simulink model "HANcoder_E407_TTA_Controller_v3_2"  (R2018b)
settings: Solver=FixedStepDiscrete  StartTime=0.0  StopTime=1  FixedStep=0.01  RelTol=1e-3
PreLoadFcn:
  | librarySetup
  | eval([bdroot,'_startup']) %Calling [modelName]_startup.m
undefined symbols (not defined in the file): A0, A1, A2, A3, A4, Backup_Board, basic_cycle_duration_bc0, basic_cycle_duration_bc1, comm_delay_estimation1, comm_delay_estimation2, COMM_Period, COMM_Phase1, COMM_Phase2, COMM_Phase_init1, COMM_Phase_init2, COMP_duration, CON2, CON4, Controller1_Board, Controller2_Board, Controller3_Board, D10, D12, D13, D8, D9, delta_a_set, delta_f_set, delta_max, delta_min, delta_precision, e_width, frequency_IRQ, HANtuneOverride, hardware_granularity, I_a, I_f, idle_time_init, Input_Gen_Board, LA_Clock_Gr, LA_COMM_dly, LA_COMM_Err, LA_E_Desync, LA_MEX_Flag, LA_Task_Act, m_v, Master_Role, matrix_cycle_duration, matrix_rows, max_desync, max_num_msgs_CAN1, max_num_msgs_CAN2, min_desync, OutControl1_ID, OutControl2_ID, OutEmulator_ID, R_al, R_ar, R_fl, R_fr ... (+80)
libraries: hdlsllib x434, HANcoder_STM32_Target x28, simulink x3, simulink_extras x1
(part 13 of 31)

== system HANcoder_E407_TTA_Controller_v3_2/HANcoder STM32 Target - E407-STM32 algorithm/TTA CAN System/TTA System/Matrix Cycle Manager/Controller Matrix Cycle/controller basic cycle 1/COMP Task - Calculate Speed/Calculate speed ==
  note: Torque range: [tau_min, tau_max]
  note: Local variables
  note: Logic Analyzer - DEBUG
      | LT Update COMP task
      | activation
  note: Logic Analyzer - DEBUG
  Enable : EnablePort
  Constant1 : Constant  Priority=28  OutDataTypeStr=boolean
  Data Store Memory43 : DataStoreMemory  DataStoreName=v_ctreff  ReadBeforeWriteMsg=warning  WriteAfterWriteMsg=warning  WriteAfterReadMsg=warning  ShowAdditionalParam=off
  Data Store Memory44 : DataStoreMemory  DataStoreName=speed_error_prev  ReadBeforeWriteMsg=warning  WriteAfterWriteMsg=warning  WriteAfterReadMsg=warning  ShowAdditionalParam=off
  Data Store Memory46 : DataStoreMemory  DataStoreName=speed_derivative  ReadBeforeWriteMsg=warning  WriteAfterWriteMsg=warning  WriteAfterReadMsg=warning  ShowAdditionalParam=off
  Data Store Read : DataStoreRead  DataStoreName=theta_dot_fr
  Data Store Read1 : DataStoreRead  DataStoreName=theta_dot_fl
  Data Store Read10 : DataStoreRead  DataStoreName=speed_integral
  Data Store Read11 : DataStoreRead  DataStoreName=speed_derivative
  Data Store Read12 : DataStoreRead  DataStoreName=torque_fr_out
  Data Store Read13 : DataStoreRead  DataStoreName=v_ctreff
  Data Store Read14 : DataStoreRead  DataStoreName=torque_fl_out
  Data Store Read15 : DataStoreRead  DataStoreName=torque_ar_out
  Data Store Read16 : DataStoreRead  DataStoreName=torque_al_out
  Data Store Read2 : DataStoreRead  DataStoreName=theta_dot_ar
  Data Store Read3 : DataStoreRead  DataStoreName=theta_dot_al
  Data Store Read4 : DataStoreRead  DataStoreName=v_est
  Data Store Read5 : DataStoreRead  DataStoreName=v_set_stored
  Data Store Read6 : DataStoreRead  DataStoreName=speed_error_prev
  Data Store Read7 : DataStoreRead  DataStoreName=rx_data_incr_time
  Data Store Read9 : DataStoreRead  DataStoreName=speed_integral
  Data Store Write : DataStoreWrite  Priority=1  DataStoreName=v_est
  Data Store Write1 : DataStoreWrite  Priority=30  DataStoreName=speed_error_prev
  Data Store Write2 : DataStoreWrite  Priority=20  DataStoreName=speed_integral
  Data Store Write3 : DataStoreWrite  Priority=21  DataStoreName=speed_derivative
  Data Store Write4 : DataStoreWrite  Priority=40  DataStoreName=v_ctreff
  Data Store Write5 : DataStoreWrite  Priority=51  DataStoreName=torque_fl_set
  Data Store Write6 : DataStoreWrite  Priority=50  DataStoreName=torque_fr_set
  Data Store Write7 : DataStoreWrite  Priority=52  DataStoreName=torque_ar_set
  Data Store Write8 : DataStoreWrite  Priority=53  DataStoreName=torque_al_set
  Data Store Write9 : DataStoreWrite  Priority=29  DataStoreName=Toggle_Pin_A0
  Derivative speed : Subsystem
  Gain : Gain  Gain=R_fr
  Gain1 : Gain  Gain=R_fl
  Gain2 : Gain  Gain=R_ar
  Gain3 : Gain  Gain=R_al
  Gain4 : Gain  Gain=1/4
  Gain5 : Gain  Gain=speed_k_p
  Gain6 : Gain  Gain=speed_k_i
  Gain7 : Gain  Gain=speed_k_d
  Integral speed : Subsystem
  Saturation{,1..3} (4 alike) : Saturate  UpperLimit=tau_max  LowerLimit=tau_min
  Saturation4 : Saturate  UpperLimit=speed_max  LowerLimit=speed_min
  Sum : Sum  Inputs=++++
  Sum1 : Sum  Priority=10  Inputs=+-
  Sum2 : Sum  Inputs=+++
  Sum{3..6} (4 alike) : Sum
  wires:
  Data Store Read/1 -> Gain/1
  Data Store Read1/1 -> Gain1/1
  Data Store Read2/1 -> Gain2/1
  Data Store Read3/1 -> Gain3/1
  Gain/1 -> Sum/1
  Gain1/1 -> Sum/2
  Gain2/1 -> Sum/3
  Gain3/1 -> Sum/4
  Sum/1 -> Gain4/1
  Gain4/1 -> Data Store Write/1  "v_est_s"
  Data Store Read5/1 -> Sum1/1
  Data Store Read4/1 -> Sum1/2
  Sum1/1 -> [v_error]
  [v_error] -> Derivative speed/1(current_value), Integral speed/2(current_value)
  Data Store Read6/1 -> Derivative speed/2(previous_value), Integral speed/3(previous_value)
  [v_error] -> Data Store Write1/1
  Data Store Read7/1 -> Derivative speed/3(incr_time), Integral speed/4(incr_time)
  Integral speed/1(result) -> Saturation4/1  "v_integral_s"
  Data Store Read9/1 -> Integral speed/1(current_integral_value)
  Derivative speed/1(result) -> Data Store Write3/1
  Gain6/1 -> Sum2/2
  Gain5/1 -> Sum2/1
  Gain7/1 -> Sum2/3
  [v_error] -> Gain5/1
  Data Store Read10/1 -> Gain6/1
  Data Store Read11/1 -> Gain7/1
  Sum2/1 -> Data Store Write4/1  "v_ctreff_s"
  Data Store Read12/1 -> Sum3/2
  Data Store Read14/1 -> Sum4/2
  Data Store Read15/1 -> Sum5/2
  Data Store Read16/1 -> Sum6/2
  Data Store Read13/1 -> Sum6/1, Sum5/1, Sum4/1, Sum3/1
  Sum4/1 -> Saturation1/1
  Sum6/1 -> Saturation3/1
  Sum5/1 -> Saturation2/1
  Sum3/1 -> Saturation/1
  Saturation/1 -> Data Store Write6/1  "torque_fr_set_s"
  Saturation1/1 -> Data Store Write5/1  "torque_fl_set_s"
  Saturation2/1 -> Data Store Write7/1  "torque_ar_set_s"
  Saturation3/1 -> Data Store Write8/1  "torque_al_set_s"
  Constant1/1 -> Data Store Write9/1
  Saturation4/1 -> Data Store Write2/1

== system HANcoder_E407_TTA_Controller_v3_2/HANcoder STM32 Target - E407-STM32 algorithm/TTA CAN System/TTA System/Matrix Cycle Manager/Controller Matrix Cycle/controller basic cycle 1/COMP Task - Calculate Steer/Calculate steering ==
  note: Local variables
  note: Logic Analyzer - DEBUG
      | LT Update COMP task
      | activation
  note: Logic Analyzer - DEBUG
  Enable : EnablePort
  Constant{,1..3} (4 alike) : Constant  Value=0
  Constant4 : Constant  Priority=28  OutDataTypeStr=boolean
  Data Store Memory23 : DataStoreMemory  DataStoreName=delta_dot_f_prev  ReadBeforeWriteMsg=warning  WriteAfterWriteMsg=warning  WriteAfterReadMsg=warning  ShowAdditionalParam=off
  Data Store Memory24 : DataStoreMemory  DataStoreName=delta_dot_a_prev  ReadBeforeWriteMsg=warning  WriteAfterWriteMsg=warning  WriteAfterReadMsg=warning  ShowAdditionalParam=off
  Data Store Read : DataStoreRead  Priority=30  DataStoreName=theta_fl_stored
  Data Store Read1 : DataStoreRead  Priority=1  DataStoreName=theta_fr_stored
  Data Store Read12 : DataStoreRead  Priority=92  DataStoreName=rx_data_incr_time
  Data Store Read16 : DataStoreRead  Priority=123  DataStoreName=rx_data_incr_time
  Data Store Read18 : DataStoreRead  Priority=153  DataStoreName=rx_data_incr_time
  Data Store Read2 : DataStoreRead  Priority=60  DataStoreName=theta_ar_stored
  Data Store Read20 : DataStoreRead  Priority=120  DataStoreName=delta_f_est
  Data Store Read21 : DataStoreRead  Priority=150  DataStoreName=delta_a_est
  Data Store Read22 : DataStoreRead  Priority=122  DataStoreName=delta_dot_f_prev
  Data Store Read23 : DataStoreRead  Priority=152  DataStoreName=delta_dot_a_prev
  Data Store Read3 : DataStoreRead  Priority=90  DataStoreName=theta_al_stored
  Data Store Read5 : DataStoreRead  Priority=3  DataStoreName=rx_data_incr_time
  Data Store Read7 : DataStoreRead  Priority=32  DataStoreName=rx_data_incr_time
  Data Store Read9 : DataStoreRead  Priority=62  DataStoreName=rx_data_incr_time
  Data Store Write : DataStoreWrite  Priority=140  DataStoreName=delta_f_est
  Data Store Write1 : DataStoreWrite  Priority=160  DataStoreName=delta_a_est
  Data Store Write2 : DataStoreWrite  Priority=142  DataStoreName=delta_dot_f_prev
  Data Store Write3 : DataStoreWrite  Priority=162  DataStoreName=delta_dot_a_prev
  Data Store Write4 : DataStoreWrite  Priority=20  DataStoreName=theta_dot_fr
  Data Store Write5 : DataStoreWrite  Priority=50  DataStoreName=theta_dot_fl
  Data Store Write6 : DataStoreWrite  Priority=80  DataStoreName=theta_dot_ar
  Data Store Write7 : DataStoreWrite  Priority=110  DataStoreName=theta_dot_al
  Data Store Write8 : DataStoreWrite  Priority=29  DataStoreName=Toggle_Pin_A0
  Derivative_theta_al : Subsystem
  Derivative_theta_ar : Subsystem
  Derivative_theta_fl : Subsystem
  Derivative_theta_fr : Subsystem
  Gain : Gain  Priority=21  Gain=R_fr
  Gain1 : Gain  Priority=51  Gain=R_fl
  Gain2 : Gain  Priority=81  Gain=R_ar
  Gain3 : Gain  Priority=111  Gain=R_al
  Gain4 : Gain  Priority=53  Gain=1/Tl_f
  Gain5 : Gain  Priority=113  Gain=1/Tl_a
  Integral_delta_a_est : Subsystem
  Integral_delta_f_est : Subsystem
  Minus : Sum  Priority=52  Inputs=+-
  Minus1 : Sum  Priority=112  Inputs=+-
  Saturation : Saturate  UpperLimit=delta_max  LowerLimit=delta_min
  Saturation1 : Saturate  UpperLimit=delta_max  LowerLimit=delta_min
  wires:
  Data Store Read1/1 -> Derivative_theta_fr/1(current_value)  "theta_fr_stored_s"
  Constant/1 -> Derivative_theta_fr/2(previous_value)
  Data Store Read5/1 -> Derivative_theta_fr/3(incr_time)
  Data Store Read7/1 -> Derivative_theta_fl/3(incr_time)
  Data Store Read9/1 -> Derivative_theta_ar/3(incr_time)
  Data Store Read12/1 -> Derivative_theta_al/3(incr_time)
  Data Store Read/1 -> Derivative_theta_fl/1(current_value)  "theta_fl_stored_s"
  Constant1/1 -> Derivative_theta_fl/2(previous_value)
  Data Store Read2/1 -> Derivative_theta_ar/1(current_value)  "theta_ar_stored_s"
  Constant2/1 -> Derivative_theta_ar/2(previous_value)
  Data Store Read3/1 -> Derivative_theta_al/1(current_value)  "theta_al_stored_s"
  Constant3/1 -> Derivative_theta_al/2(previous_value)
  Derivative_theta_fr/1(result) -> Gain/1, Data Store Write4/1
  Derivative_theta_ar/1(result) -> Gain2/1, Data Store Write6/1
  Derivative_theta_al/1(result) -> Data Store Write7/1, Gain3/1
  Gain/1 -> Minus/1
  Gain1/1 -> Minus/2
  Gain2/1 -> Minus1/1
  Gain3/1 -> Minus1/2
  Minus/1 -> Gain4/1
  Minus1/1 -> Gain5/1
  Gain4/1 -> [delta_dot_f]
  Integral_delta_f_est/1(result) -> Saturation/1
  Gain5/1 -> [delta_dot_a]
  Integral_delta_a_est/1(result) -> Saturation1/1
  Data Store Read16/1 -> Integral_delta_f_est/4(incr_time)
  Data Store Read20/1 -> Integral_delta_f_est/1(current_integral_value)
  Data Store Read18/1 -> Integral_delta_a_est/4(incr_time)
  Data Store Read21/1 -> Integral_delta_a_est/1(current_integral_value)
  Data Store Read22/1 -> Integral_delta_f_est/3(previous_value)
  Data Store Read23/1 -> Integral_delta_a_est/3(previous_value)
  [delta_dot_a] -> Data Store Write3/1
  [delta_dot_f] -> Data Store Write2/1
  Derivative_theta_fl/1(result) -> Gain1/1, Data Store Write5/1
  [delta_dot_f] -> Integral_delta_f_est/2(current_value)
  [delta_dot_a] -> Integral_delta_a_est/2(current_value)
  Constant4/1 -> Data Store Write8/1
  Saturation/1 -> Data Store Write/1
  Saturation1/1 -> Data Store Write1/1

== system HANcoder_E407_TTA_Controller_v3_2/HANcoder STM32 Target - E407-STM32 algorithm/TTA CAN System/TTA System/Matrix Cycle Manager/Controller Matrix Cycle/controller basic cycle 1/COMP Task - Calculate Torque/Calculate torque ==
  note: Local variables
  note: Logic Analyzer - DEBUG
      | LT Update COMP task
      | activation
  note: Logic Analyzer - DEBUG
  Enable : EnablePort
  Constant1 : Constant  Priority=28  OutDataTypeStr=boolean
  Data Store Memory27 : DataStoreMemory  DataStoreName=delta_f_error_prev  ReadBeforeWriteMsg=warning  WriteAfterWriteMsg=warning  WriteAfterReadMsg=warning  ShowAdditionalParam=off
  Data Store Memory28 : DataStoreMemory  DataStoreName=delta_a_error_prev  ReadBeforeWriteMsg=warning  WriteAfterWriteMsg=warning  WriteAfterReadMsg=warning  ShowAdditionalParam=off
  Data Store Memory30 : DataStoreMemory  DataStoreName=torque_fr_derivative  ReadBeforeWriteMsg=warning  WriteAfterWriteMsg=warning  WriteAfterReadMsg=warning  ShowAdditionalParam=off
  Data Store Memory33 : DataStoreMemory  DataStoreName=torque_ar_derivative  ReadBeforeWriteMsg=warning  WriteAfterWriteMsg=warning  WriteAfterReadMsg=warning  ShowAdditionalParam=off
  Data Store Read : DataStoreRead  DataStoreName=torque_fr_out
  Data Store Read1 : DataStoreRead  DataStoreName=torque_ar_out
  Data Store Read10 : DataStoreRead  DataStoreName=torque_ar_integral
  Data Store Read11 : DataStoreRead  DataStoreName=delta_a_error_prev
  Data Store Read12 : DataStoreRead  DataStoreName=torque_fr_integral
  Data Store Read13 : DataStoreRead  DataStoreName=torque_fr_derivative
  Data Store Read14 : DataStoreRead  DataStoreName=torque_ar_integral
  Data Store Read15 : DataStoreRead  DataStoreName=torque_ar_derivative
  Data Store Read2 : DataStoreRead  Priority=1  DataStoreName=delta_f_set_stored
  Data Store Read3 : DataStoreRead  Priority=2  DataStoreName=delta_f_est
  Data Store Read4 : DataStoreRead  Priority=4  DataStoreName=delta_a_set_stored
  Data Store Read5 : DataStoreRead  Priority=5  DataStoreName=delta_a_est
  Data Store Read6 : DataStoreRead  DataStoreName=rx_data_incr_time
  Data Store Read8 : DataStoreRead  DataStoreName=torque_fr_integral
  Data Store Read9 : DataStoreRead  DataStoreName=delta_f_error_prev
  Data Store Write : DataStoreWrite  Priority=30  DataStoreName=torque_fr_out
  Data Store Write1 : DataStoreWrite  Priority=40  DataStoreName=torque_fl_out
  Data Store Write10 : DataStoreWrite  Priority=29  DataStoreName=Toggle_Pin_A0
  Data Store Write2 : DataStoreWrite  Priority=31  DataStoreName=torque_ar_out
  Data Store Write3 : DataStoreWrite  Priority=41  DataStoreName=torque_al_out
  Data Store Write4 : DataStoreWrite  Priority=10  DataStoreName=torque_fr_integral
  Data Store Write5 : DataStoreWrite  Priority=20  DataStoreName=delta_f_error_prev
  Data Store Write6 : DataStoreWrite  Priority=11  DataStoreName=torque_fr_derivative
  Data Store Write7 : DataStoreWrite  Priority=12  DataStoreName=torque_ar_integral
  Data Store Write8 : DataStoreWrite  Priority=13  DataStoreName=torque_ar_derivative
  Data Store Write9 : DataStoreWrite  Priority=21  DataStoreName=delta_a_error_prev
  Derivative torque aft : Subsystem
  Derivative torque front : Subsystem
  Gain : Gain  Gain=-1
  Gain1 : Gain  Gain=-1
  Gain2 : Gain  Gain=torque_f_k_p
  Gain3 : Gain  Gain=torque_f_k_i
  Gain4 : Gain  Gain=torque_f_k_d
  Gain5 : Gain  Gain=torque_a_k_p
  Gain6 : Gain  Gain=torque_a_k_i
  Gain7 : Gain  Gain=torque_a_k_d
  Integral torque aft : Subsystem
  Integral_torque_front : Subsystem
  Minus : Sum  Priority=3  Inputs=+-
  Minus1 : Sum  Priority=6  Inputs=+-
  Saturation : Saturate  UpperLimit=tau_max  LowerLimit=tau_min
  Saturation1 : Saturate  UpperLimit=tau_max  LowerLimit=tau_min
  Sum : Sum  Inputs=+++
  Sum1 : Sum  Inputs=+++
  wires:
  Integral_torque_front/1(result) -> Saturation/1
  Derivative torque front/1(result) -> Data Store Write6/1
  Data Store Read/1 -> Gain/1
  Sum/1 -> Data Store Write/1
  Data Store Read1/1 -> Gain1/1
  Sum1/1 -> Data Store Write2/1
  Derivative torque aft/1(result) -> Data Store Write8/1
  Integral torque aft/1(result) -> Saturation1/1
  Data Store Read2/1 -> Minus/1
  Data Store Read3/1 -> Minus/2
  Data Store Read5/1 -> Minus1/2
  Data Store Read4/1 -> Minus1/1
  [delta_f_error] -> Integral_torque_front/2(current_value), Derivative torque front/1(current_value)
  [delta_a_error] -> Derivative torque aft/1(current_value), Integral torque aft/2(current_value)
  Data Store Read6/1 -> Integral_torque_front/4(incr_time), Derivative torque aft/3(incr_time), Integral torque aft/4(incr_time), Derivative torque front/3(incr_time)
  Gain/1 -> Data Store Write1/1
  Gain1/1 -> Data Store Write3/1
  Data Store Read8/1 -> Integral_torque_front/1(current_integral_value)
  Data Store Read9/1 -> Integral_torque_front/3(previous_value), Derivative torque front/2(previous_value)
  Minus/1 -> [delta_f_error]
  [delta_f_error] -> Data Store Write5/1
  Minus1/1 -> [delta_a_error]
  Data Store Read10/1 -> Integral torque aft/1(current_integral_value)
  Data Store Read11/1 -> Derivative torque aft/2(previous_value), Integral torque aft/3(previous_value)
  [delta_a_error] -> Data Store Write9/1
  [delta_f_error] -> Gain2/1
  Gain2/1 -> Sum/1
  Gain3/1 -> Sum/2
  Gain4/1 -> Sum/3
  Data Store Read12/1 -> Gain3/1
  Data Store Read13/1 -> Gain4/1
  Data Store Read15/1 -> Gain7/1
  Data Store Read14/1 -> Gain6/1
  Gain7/1 -> Sum1/3
  Gain6/1 -> Sum1/2
  Gain5/1 -> Sum1/1
  [delta_a_error] -> Gain5/1
  Constant1/1 -> Data Store Write10/1
  Saturation/1 -> Data Store Write4/1
  Saturation1/1 -> Data Store Write7/1

== system HANcoder_E407_TTA_Controller_v3_2/HANcoder STM32 Target - E407-STM32 algorithm/TTA CAN System/TTA System/Matrix Cycle Manager/Controller Matrix Cycle/controller basic cycle 1/COMP Task - Reset Variables BC1/Check Timeouts ==
  note: Timeout Master counter
  note: Set values missed counter
  note: Sensor values missed counter
  note: Output Controller 1 missed counter
  note: Output Controller 2 missed counter
  note: Logic Analyzer - DEBUG
  note: Logic Analyzer - DEBUG
      | Increase Error counter
  Enable : EnablePort
  AND1 : Logic  IconShape=distinctive  AllPortsSameDT=off  OutDataTypeStr=boolean
  AND2 : Logic  IconShape=distinctive  AllPortsSameDT=off  OutDataTypeStr=boolean
  AND9 : Logic  IconShape=distinctive  AllPortsSameDT=off  OutDataTypeStr=boolean
  Constant{1..4,16} (5 alike) : Constant
  Data Store Read1 : DataStoreRead  DataStoreName=Set_missed_counter
  Data Store Read10 : DataStoreRead  DataStoreName=Out2_missed_counter
  Data Store Read11 : DataStoreRead  DataStoreName=Out2_missed_counter
  Data Store Read12 : DataStoreRead  DataStoreName=Master_ID
  Data Store Read13 : DataStoreRead  DataStoreName=Master_ID
  Data Store Read14 : DataStoreRead  DataStoreName=Board_ID
  Data Store Read15 : DataStoreRead  DataStoreName=Board_ID
  Data Store Read16 : DataStoreRead  DataStoreName=output_control2_rx
  Data Store Read2 : DataStoreRead  DataStoreName=Set_missed_counter
  Data Store Read23 : DataStoreRead  DataStoreName=Sync_bc1_missed_counter
  Data Store Read24 : DataStoreRead  DataStoreName=Sync_bc1_missed_counter
  Data Store Read25 : DataStoreRead  DataStoreName=BC1_Sync_processed
  Data Store Read26 : DataStoreRead  DataStoreName=Master_ID
  Data Store Read27 : DataStoreRead  DataStoreName=Board_ID
  Data Store Read3 : DataStoreRead  DataStoreName=Error_SetValues_NotRX
  Data Store Read4 : DataStoreRead  DataStoreName=Sensor_missed_counter
  Data Store Read5 : DataStoreRead  DataStoreName=Sensor_missed_counter
  Data Store Read6 : DataStoreRead  DataStoreName=Error_SensorValues_NotRX
  Data Store Read7 : DataStoreRead  DataStoreName=Out1_missed_counter
  Data Store Read8 : DataStoreRead  DataStoreName=Out1_missed_counter
  Data Store Read9 : DataStoreRead  DataStoreName=output_control1_rx
  Data Store Write1 : DataStoreWrite  DataStoreName=Set_missed_counter
  Data Store Write2 : DataStoreWrite  DataStoreName=Sensor_missed_counter
  Data Store Write3 : DataStoreWrite  DataStoreName=Out1_missed_counter
  Data Store Write4 : DataStoreWrite  DataStoreName=Out2_missed_counter
  Data Store Write8 : DataStoreWrite  DataStoreName=Toggle_Pin_A1
  Data Store Write9 : DataStoreWrite  DataStoreName=Sync_bc1_missed_counter
  Equal1 : RelationalOperator  Operator===  OutDataTypeStr=boolean  RndMeth=Simplest
  Equal2 : RelationalOperator  Operator===  OutDataTypeStr=boolean  RndMeth=Simplest
  Equal9 : RelationalOperator  Operator=~=  OutDataTypeStr=boolean  RndMeth=Simplest
  NOT : Logic  Operator=NOT  IconShape=distinctive  AllPortsSameDT=off  OutDataTypeStr=boolean
  NOT1 : Logic  Operator=NOT  IconShape=distinctive  AllPortsSameDT=off  OutDataTypeStr=boolean
  NOT4 : Logic  Operator=NOT  IconShape=distinctive  AllPortsSameDT=off  OutDataTypeStr=boolean
  OR : Logic  Operator=OR  Inputs=5  IconShape=distinctive  AllPortsSameDT=off  OutDataTypeStr=boolean
  Plus{1..4,6} (5 alike) : Sum
  Switch{1..4,7} (5 alike) : Switch  Criteria=u2 > Threshold
  wires:
  Constant16/1 -> Plus6/2
  Data Store Read23/1 -> Plus6/1
  NOT4/1 -> AND9/1
  Data Store Read24/1 -> Switch7/3
  Data Store Read25/1 -> NOT4/1
  Data Store Read26/1 -> Equal9/1
  Data Store Read27/1 -> Equal9/2
  Equal9/1 -> AND9/2
  Plus6/1 -> Switch7/1
  Switch7/1 -> Data Store Write9/1
  AND9/1 -> [increase_sync], Switch7/2
  Data Store Read3/1 -> [increase_set], Switch1/2
  Switch1/1 -> Data Store Write1/1
  Plus1/1 -> Switch1/1
  Data Store Read2/1 -> Switch1/3
  Data Store Read1/1 -> Plus1/1
  Constant1/1 -> Plus1/2
  Constant2/1 -> Plus2/2
  Data Store Read4/1 -> Plus2/1
  Data Store Read5/1 -> Switch2/3
  Plus2/1 -> Switch2/1
  Switch2/1 -> Data Store Write2/1
  Data Store Read6/1 -> [increase_sensor], Switch2/2
  Data Store Read9/1 -> NOT/1
  Switch3/1 -> Data Store Write3/1
  Plus3/1 -> Switch3/1
  Data Store Read8/1 -> Switch3/3
  Data Store Read7/1 -> Plus3/1
  Constant3/1 -> Plus3/2
  AND1/1 -> [increase_out1], Switch3/2
  AND2/1 -> [increase_out2], Switch4/2
  Constant4/1 -> Plus4/2
  Data Store Read10/1 -> Plus4/1
  Data Store Read11/1 -> Switch4/3
  Plus4/1 -> Switch4/1
  Switch4/1 -> Data Store Write4/1
  [increase_set] -> OR/2
  [increase_out1] -> OR/4
  [increase_out2] -> OR/5
  OR/1 -> Data Store Write8/1
  [increase_sync] -> OR/1
  [increase_sensor] -> OR/3
  Equal1/1 -> AND1/2
  Data Store Read14/1 -> Equal1/2
  Data Store Read13/1 -> Equal1/1
  NOT/1 -> AND1/1
  NOT1/1 -> AND2/1
  Data Store Read12/1 -> Equal2/1
  Equal2/1 -> AND2/2
  Data Store Read16/1 -> NOT1/1
  Data Store Read15/1 -> Equal2/2

== system HANcoder_E407_TTA_Controller_v3_2/HANcoder STM32 Target - E407-STM32 algorithm/TTA CAN System/TTA System/Matrix Cycle Manager/Controller Matrix Cycle/controller basic cycle 1/COMP Task - Reset Variables BC1/Reset Variables ==
  note: Reset variables
  note: Logic Analyzer - DEBUG
      | Start of COMP task
  note: Logic Analyzer - DEBUG
  Enable : EnablePort
  Constant : Constant  Value=0  OutDataTypeStr=boolean
  Constant3 : Constant  OutDataTypeStr=boolean
  Data Store Write : DataStoreWrite  DataStoreName=Desync_Positive
  Data Store Write1 : DataStoreWrite  DataStoreName=BC1_Sync_processed
  Data Store Write3 : DataStoreWrite  DataStoreName=Toggle_Pin_A0
  wires:
  Constant/1 -> Data Store Write/1, Data Store Write1/1
  Constant3/1 -> Data Store Write3/1

== system HANcoder_E407_TTA_Controller_v3_2/HANcoder STM32 Target - E407-STM32 algorithm/TTA CAN System/TTA System/Matrix Cycle Manager/Controller Matrix Cycle/controller basic cycle 1/COMP Task - Rx_Output_Control1_Check/OutputControl1 Tx condition ==
  note: During Ouput Controller 1 only boards
      | 1 or 2 are going to transmit. If the master
      | (this board) is Board 1, then the msg was
      | transmitted from Board 2. Otherwise, the
      | msg was transmitted from Board 1.
  note: During Ouput Controller 1 and Output Controller 2
      | the slaves send information to the master about
      | their torque calculations. The slave with lowest ID
      | will transmit first. This means that if Board 1 is a
      | a slave, it is always going to transmit during
      | Output Controller 1, and if Board 3 is a slave, it is
      | always going to transmit during Output Controller 2.
      | Board number 2 will transmit during one COMM or
      | the other depending on who is the master board
      | for this basic cycle.
  Constant4 : Constant
  Constant5 : Constant  Value=2
  Constant8 : Constant
  Data Store Read3 : DataStoreRead  DataStoreName=Board_ID
  Equal4 : RelationalOperator  Operator===  OutDataTypeStr=boolean  RndMeth=Simplest
  Switch : Switch  Criteria=u2 > Threshold
  Out1 : Outport
  wires:
  Switch/1 -> Out1/1
  Equal4/1 -> Switch/2
  Data Store Read3/1 -> Equal4/1
  Constant4/1 -> Equal4/2
  Constant5/1 -> Switch/1
  Constant8/1 -> Switch/3

== system HANcoder_E407_TTA_Controller_v3_2/HANcoder STM32 Target - E407-STM32 algorithm/TTA CAN System/TTA System/Matrix Cycle Manager/Controller Matrix Cycle/controller basic cycle 1/COMP Task - Rx_Output_Control1_Check/Process_Messages ==
  note: Logic Analyzer - DEBUG
  note: Logic Analyzer - DEBUG
      | Sync_Check COMP task
      | activation
  new_CAN1_msg : Inport
  new_CAN2_msg : Inport  Port=2
  Rx_msg_CAN1 : Inport  Port=3  OutDataTypeStr=Bus: msg_buffer_type
  Rx_Msg_CAN2 : Inport  Port=4  OutDataTypeStr=Bus: msg_buffer_type
  expected_board_id : Inport  Port=5
  Enable : EnablePort
  Bus Selector : BusSelector  OutputSignals=signal1,Buffer_2,Buffer_3,Buffer_4,Buffer_5,Buffer_6,Buffer_7,Buffer_8
  Constant2 : Constant  Priority=28  OutDataTypeStr=boolean
  Data Store Write : DataStoreWrite  Priority=4  DataStoreName=output_control1_msg  DataStoreElements=output_control1_msg.Buffer_1#output_control1_msg.Buffer_2#output_control1_msg.Buffer_3#output_control1_msg.Buffer_4#output_control1_msg.Buffer_5#output_control1_msg.Buffer_6#output_control1_msg.Buffer_7#output_control1_msg.Buffer_8
  Data Store Write3 : DataStoreWrite  Priority=29  DataStoreName=Toggle_Pin_A0
  Data Store Write4 : DataStoreWrite  DataStoreName=output_control1_rx
  Demux message CAN1 and check coherence : Subsystem  Priority=1
  Demux message CAN1 and check coherence1 : Subsystem  Priority=2
  OR : Logic  Operator=OR  IconShape=distinctive  AllPortsSameDT=off  OutDataTypeStr=boolean
  Switch : Switch  Priority=3  Criteria=u2 > Threshold
  Terminator : Terminator
  Terminator1 : Terminator
  wires:
  Bus Selector/2 -> Data Store Write/2  "<Buffer_2>"
  Bus Selector/6 -> Data Store Write/6  "<Buffer_6>"
  Switch/1 -> Bus Selector/1
  Bus Selector/8 -> Data Store Write/8  "<Buffer_8>"
  Bus Selector/1 -> Data Store Write/1  "<signal1>"
  Bus Selector/7 -> Data Store Write/7  "<Buffer_7>"
  Bus Selector/4 -> Data Store Write/4  "<Buffer_4>"
  Bus Selector/3 -> Data Store Write/3  "<Buffer_3>"
  Bus Selector/5 -> Data Store Write/5  "<Buffer_5>"
  Demux message CAN1 and check coherence1/2(Msg_Count_CAN2) -> Terminator/1
  Demux message CAN1 and check coherence/2(Msg_Count_CAN1) -> Terminator1/1
  expected_board_id/1 -> Demux message CAN1 and check coherence1/2(expected_board_id), Demux message CAN1 and check coherence/2(expected_board_id)
  Constant2/1 -> Data Store Write3/1
  OR/1 -> Data Store Write4/1  "out1_rx_s"
  Demux message CAN1 and check coherence1/3(CAN2_msg) -> Switch/3
  Demux message CAN1 and check coherence1/1(CAN2_msg_coherent) -> OR/2
  Demux message CAN1 and check coherence/1(CAN1_msg) -> Switch/1
  Demux message CAN1 and check coherence/3(CAN1_msg_coherent) -> OR/1, Switch/2
  Rx_Msg_CAN2/1 -> Demux message CAN1 and check coherence1/1(CAN2_Rx_msg)
  Rx_msg_CAN1/1 -> Demux message CAN1 and check coherence/1(CAN1_Rx_msg)
  new_CAN2_msg/1 -> Demux message CAN1 and check coherence1/Enable
  new_CAN1_msg/1 -> Demux message CAN1 and check coherence/Enable

== system HANcoder_E407_TTA_Controller_v3_2/HANcoder STM32 Target - E407-STM32 algorithm/TTA CAN System/TTA System/Matrix Cycle Manager/Controller Matrix Cycle/controller basic cycle 1/COMP Task - Rx_Output_Control1_Check/Reset Tx msg counter ==
  Enable : EnablePort
  Constant1 : Constant  Priority=2
  Constant6 : Constant  Priority=2
  Data Store Write1 : DataStoreWrite  Priority=4  DataStoreName=Tx_msg_count_CAN1
  Data Store Write2 : DataStoreWrite  Priority=4  DataStoreName=Tx_msg_count_CAN2
  wires:
  Constant1/1 -> Data Store Write2/1
  Constant6/1 -> Data Store Write1/1

== system HANcoder_E407_TTA_Controller_v3_2/HANcoder STM32 Target - E407-STM32 algorithm/TTA CAN System/TTA System/Matrix Cycle Manager/Controller Matrix Cycle/controller basic cycle 1/COMP Task - Rx_Output_Control2_Check/OutputControl1 Tx condition2 ==
  note: During Ouput Controller 2 only boards
      | 2 or 3 are going to transmit. If the master
      | (this board) is Board 3, then the msg was
      | transmitted from Board 2. Otherwise, the
      | msg was transmitted from Board 3.
  note: During Ouput Controller 1 and Output Controller 2
      | the slaves send information to the master about
      | their torque calculations. The slave with lowest ID
      | will transmit first. This means that if Board 1 is a
      | a slave, it is always going to transmit during
      | Output Controller 1, and if Board 3 is a slave, it is
      | always going to transmit during Output Controller 2.
      | Board number 2 will transmit during one COMM or
      | the other depending on who is the master board
      | for this basic cycle.
  Constant4 : Constant  Value=3
  Constant5 : Constant  Value=2
  Constant8 : Constant  Value=3
  Data Store Read3 : DataStoreRead  DataStoreName=Board_ID
  Equal4 : RelationalOperator  Operator===  OutDataTypeStr=boolean  RndMeth=Simplest
  Switch : Switch  Criteria=u2 > Threshold
  Tx_Board_ID_Out2 : Outport
  wires:
  Switch/1 -> Tx_Board_ID_Out2/1
  Equal4/1 -> Switch/2
  Data Store Read3/1 -> Equal4/1
  Constant4/1 -> Equal4/2
  Constant5/1 -> Switch/1
  Constant8/1 -> Switch/3

== system HANcoder_E407_TTA_Controller_v3_2/HANcoder STM32 Target - E407-STM32 algorithm/TTA CAN System/TTA System/Matrix Cycle Manager/Controller Matrix Cycle/controller basic cycle 1/COMP Task - Rx_Output_Control2_Check/Process_Messages ==
  note: Logic Analyzer - DEBUG
      | Sync_Check COMP task
      | activation
  note: Logic Analyzer - DEBUG
  new_CAN1_msg : Inport
  new_CAN2_msg : Inport  Port=2
  Rx_msg_CAN1 : Inport  Port=3  OutDataTypeStr=Bus: msg_buffer_type
  Rx_Msg_CAN2 : Inport  Port=4  OutDataTypeStr=Bus: msg_buffer_type
  expected_board_id : Inport  Port=5
  Enable : EnablePort
  Bus Selector : BusSelector  OutputSignals=signal1,Buffer_2,Buffer_3,Buffer_4,Buffer_5,Buffer_6,Buffer_7,Buffer_8
  Constant2 : Constant  Priority=28  OutDataTypeStr=boolean
  Data Store Write : DataStoreWrite  Priority=4  DataStoreName=output_control2_msg  DataStoreElements=output_control2_msg.Buffer_1#output_control2_msg.Buffer_2#output_control2_msg.Buffer_3#output_control2_msg.Buffer_4#output_control2_msg.Buffer_5#output_control2_msg.Buffer_6#output_control2_msg.Buffer_7#output_control2_msg.Buffer_8
  Data Store Write3 : DataStoreWrite  Priority=29  DataStoreName=Toggle_Pin_A0
  Data Store Write4 : DataStoreWrite  DataStoreName=output_control2_rx
  Demux message CAN1 and check coherence : Subsystem  Priority=1
  Demux message CAN1 and check coherence1 : Subsystem  Priority=2
  OR : Logic  Operator=OR  IconShape=distinctive  AllPortsSameDT=off  OutDataTypeStr=boolean
  Switch : Switch  Priority=3  Criteria=u2 > Threshold
  Terminator : Terminator
  Terminator1 : Terminator
  wires:
  new_CAN1_msg/1 -> Demux message CAN1 and check coherence/Enable
  new_CAN2_msg/1 -> Demux message CAN1 and check coherence1/Enable
  Rx_msg_CAN1/1 -> Demux message CAN1 and check coherence/1(CAN1_Rx_msg)
  Rx_Msg_CAN2/1 -> Demux message CAN1 and check coherence1/1(CAN2_Rx_msg)
  Demux message CAN1 and check coherence/3(CAN1_msg_coherent) -> Switch/2, OR/1
  Demux message CAN1 and check coherence/1(CAN1_msg) -> Switch/1
  Demux message CAN1 and check coherence1/1(CAN2_msg_coherent) -> OR/2
  Demux message CAN1 and check coherence1/3(CAN2_msg) -> Switch/3
  OR/1 -> Data Store Write4/1  "out2_rx_s"
  Constant2/1 -> Data Store Write3/1
  expected_board_id/1 -> Demux message CAN1 and check coherence/2(expected_board_id), Demux message CAN1 and check coherence1/2(expected_board_id)
  Demux message CAN1 and check coherence/2(Msg_Count_CAN1) -> Terminator/1
  Demux message CAN1 and check coherence1/2(Msg_Count_CAN2) -> Terminator1/1
  Bus Selector/5 -> Data Store Write/5  "<Buffer_5>"
  Bus Selector/3 -> Data Store Write/3  "<Buffer_3>"
  Bus Selector/4 -> Data Store Write/4  "<Buffer_4>"
  Bus Selector/7 -> Data Store Write/7  "<Buffer_7>"
  Bus Selector/1 -> Data Store Write/1  "<signal1>"
  Bus Selector/8 -> Data Store Write/8  "<Buffer_8>"
  Switch/1 -> Bus Selector/1
  Bus Selector/6 -> Data Store Write/6  "<Buffer_6>"
  Bus Selector/2 -> Data Store Write/2  "<Buffer_2>"

== system HANcoder_E407_TTA_Controller_v3_2/HANcoder STM32 Target - E407-STM32 algorithm/TTA CAN System/TTA System/Matrix Cycle Manager/Controller Matrix Cycle/controller basic cycle 1/COMP Task - Rx_Output_Control2_Check/Reset Tx msg counter ==
  Enable : EnablePort
  Constant1 : Constant  Priority=2
  Constant6 : Constant  Priority=2
  Data Store Write1 : DataStoreWrite  Priority=4  DataStoreName=Tx_msg_count_CAN1
  Data Store Write2 : DataStoreWrite  Priority=4  DataStoreName=Tx_msg_count_CAN2
  wires:
  Constant6/1 -> Data Store Write1/1
  Constant1/1 -> Data Store Write2/1

== system HANcoder_E407_TTA_Controller_v3_2/HANcoder STM32 Target - E407-STM32 algorithm/TTA CAN System/TTA System/Matrix Cycle Manager/Controller Matrix Cycle/controller basic cycle 1/COMP Task - Rx_Output_Emulator_Check/Process_Messages ==
  note: Logic Analyzer - DEBUG
  note: Logic Analyzer - DEBUG
      | Sync_Check COMP task
      | activation
  new_CAN1_msg : Inport
  new_CAN2_msg : Inport  Port=2
  Rx_msg_CAN1 : Inport  Port=3  OutDataTypeStr=Bus: msg_buffer_type
  Rx_Msg_CAN2 : Inport  Port=4  OutDataTypeStr=Bus: msg_buffer_type
  expected_board_id : Inport  Port=5
  Enable : EnablePort
  Bus Selector : BusSelector  OutputSignals=signal1,Buffer_2,Buffer_3,Buffer_4,Buffer_5,Buffer_6,Buffer_7,Buffer_8
  Constant2 : Constant  Priority=28  OutDataTypeStr=boolean
  Data Store Write : DataStoreWrite  Priority=4  DataStoreName=Msg_Rx  DataStoreElements=Msg_Rx.Buffer_1#Msg_Rx.Buffer_2#Msg_Rx.Buffer_3#Msg_Rx.Buffer_4#Msg_Rx.Buffer_5#Msg_Rx.Buffer_6#Msg_Rx.Buffer_7#Msg_Rx.Buffer_8
  Data Store Write2 : DataStoreWrite  DataStoreName=new_msg_Rx
  Data Store Write3 : DataStoreWrite  Priority=29  DataStoreName=Toggle_Pin_A0
  Demux message CAN1 and check coherence : Subsystem  Priority=1
  Demux message CAN1 and check coherence1 : Subsystem  Priority=2
  OR : Logic  Operator=OR  IconShape=distinctive  AllPortsSameDT=off  OutDataTypeStr=boolean
  Switch : Switch  Priority=3  Criteria=u2 > Threshold
  Terminator : Terminator
  Terminator1 : Terminator
  wires:
  Bus Selector/2 -> Data Store Write/2  "<Buffer_2>"
  Bus Selector/6 -> Data Store Write/6  "<Buffer_6>"
  Switch/1 -> Bus Selector/1
  Bus Selector/8 -> Data Store Write/8  "<Buffer_8>"
  Bus Selector/1 -> Data Store Write/1  "<signal1>"
  Bus Selector/7 -> Data Store Write/7  "<Buffer_7>"
  Bus Selector/4 -> Data Store Write/4  "<Buffer_4>"
  Bus Selector/3 -> Data Store Write/3  "<Buffer_3>"
  Bus Selector/5 -> Data Store Write/5  "<Buffer_5>"
  Demux message CAN1 and check coherence1/2(Msg_Count_CAN2) -> Terminator/1
  Demux message CAN1 and check coherence/2(Msg_Count_CAN1) -> Terminator1/1
  expected_board_id/1 -> Demux message CAN1 and check coherence1/2(expected_board_id), Demux message CAN1 and check coherence/2(expected_board_id)
  Constant2/1 -> Data Store Write3/1
  OR/1 -> Data Store Write2/1
  Demux message CAN1 and check coherence1/3(CAN2_msg) -> Switch/3
  Demux message CAN1 and check coherence1/1(CAN2_msg_coherent) -> OR/2
  Demux message CAN1 and check coherence/1(CAN1_msg) -> Switch/1
  Demux message CAN1 and check coherence/3(CAN1_msg_coherent) -> OR/1, Switch/2
  Rx_Msg_CAN2/1 -> Demux message CAN1 and check coherence1/1(CAN2_Rx_msg)
  Rx_msg_CAN1/1 -> Demux message CAN1 and check coherence/1(CAN1_Rx_msg)
  new_CAN2_msg/1 -> Demux message CAN1 and check coherence1/Enable
  new_CAN1_msg/1 -> Demux message CAN1 and check coherence/Enable

== system HANcoder_E407_TTA_Controller_v3_2/HANcoder STM32 Target - E407-STM32 algorithm/TTA CAN System/TTA System/Matrix Cycle Manager/Controller Matrix Cycle/controller basic cycle 1/COMP Task - Rx_Output_Emulator_Check/Reset Tx msg counter ==
  Enable : EnablePort
  Constant1 : Constant  Priority=2
  Constant6 : Constant  Priority=2
  Data Store Write1 : DataStoreWrite  Priority=4  DataStoreName=Tx_msg_count_CAN1
  Data Store Write2 : DataStoreWrite  Priority=4  DataStoreName=Tx_msg_count_CAN2
  wires:
  Constant1/1 -> Data Store Write2/1
  Constant6/1 -> Data Store Write1/1

== system HANcoder_E407_TTA_Controller_v3_2/HANcoder STM32 Target - E407-STM32 algorithm/TTA CAN System/TTA System/Matrix Cycle Manager/Controller Matrix Cycle/controller basic cycle 1/COMP Task - Rx_Sensor_Values_Check/Process_Messages ==
  note: Logic Analyzer - DEBUG
      | Sync_Check COMP task
      | activation
  note: Logic Analyzer - DEBUG
  new_CAN1_msg : Inport
  new_CAN2_msg : Inport  Port=2
  Rx_msg_CAN1 : Inport  Port=3  OutDataTypeStr=Bus: msg_buffer_type
  Rx_Msg_CAN2 : Inport  Port=4  OutDataTypeStr=Bus: msg_buffer_type
  expected_board_id : Inport  Port=5
  Enable : EnablePort
  Bus Selector : BusSelector  OutputSignals=signal1,Buffer_2,Buffer_3,Buffer_4,Buffer_5,Buffer_6,Buffer_7,Buffer_8
  Constant2 : Constant  Priority=28  OutDataTypeStr=boolean
  Data Store Write : DataStoreWrite  Priority=4  DataStoreName=Msg_Rx  DataStoreElements=Msg_Rx.Buffer_1#Msg_Rx.Buffer_2#Msg_Rx.Buffer_3#Msg_Rx.Buffer_4#Msg_Rx.Buffer_5#Msg_Rx.Buffer_6#Msg_Rx.Buffer_7#Msg_Rx.Buffer_8
  Data Store Write2 : DataStoreWrite  DataStoreName=new_msg_Rx
  Data Store Write3 : DataStoreWrite  Priority=29  DataStoreName=Toggle_Pin_A0
  Demux message CAN1 and check coherence : Subsystem  Priority=1
  Demux message CAN1 and check coherence1 : Subsystem  Priority=2
  OR : Logic  Operator=OR  IconShape=distinctive  AllPortsSameDT=off  OutDataTypeStr=boolean
  Switch : Switch  Priority=3  Criteria=u2 > Threshold
  Terminator : Terminator
  Terminator1 : Terminator
  wires:
  new_CAN1_msg/1 -> Demux message CAN1 and check coherence/Enable
  new_CAN2_msg/1 -> Demux message CAN1 and check coherence1/Enable
  Rx_msg_CAN1/1 -> Demux message CAN1 and check coherence/1(CAN1_Rx_msg)
  Rx_Msg_CAN2/1 -> Demux message CAN1 and check coherence1/1(CAN2_Rx_msg)
  Demux message CAN1 and check coherence/3(CAN1_msg_coherent) -> Switch/2, OR/1
  Demux message CAN1 and check coherence/1(CAN1_msg) -> Switch/1
  Demux message CAN1 and check coherence1/1(CAN2_msg_coherent) -> OR/2
  Demux message CAN1 and check coherence1/3(CAN2_msg) -> Switch/3
  OR/1 -> Data Store Write2/1
  Constant2/1 -> Data Store Write3/1
  expected_board_id/1 -> Demux message CAN1 and check coherence/2(expected_board_id), Demux message CAN1 and check coherence1/2(expected_board_id)
  Demux message CAN1 and check coherence/2(Msg_Count_CAN1) -> Terminator/1
  Demux message CAN1 and check coherence1/2(Msg_Count_CAN2) -> Terminator1/1
  Bus Selector/5 -> Data Store Write/5  "<Buffer_5>"
  Bus Selector/3 -> Data Store Write/3  "<Buffer_3>"
  Bus Selector/4 -> Data Store Write/4  "<Buffer_4>"
  Bus Selector/7 -> Data Store Write/7  "<Buffer_7>"
  Bus Selector/1 -> Data Store Write/1  "<signal1>"
  Bus Selector/8 -> Data Store Write/8  "<Buffer_8>"
  Bus Selector/6 -> Data Store Write/6  "<Buffer_6>"
  Bus Selector/2 -> Data Store Write/2  "<Buffer_2>"
  Switch/1 -> Bus Selector/1

== system HANcoder_E407_TTA_Controller_v3_2/HANcoder STM32 Target - E407-STM32 algorithm/TTA CAN System/TTA System/Matrix Cycle Manager/Controller Matrix Cycle/controller basic cycle 1/COMP Task - Rx_Sensor_Values_Check/Reset Tx msg counter ==
  Enable : EnablePort
  Constant1 : Constant  Priority=2
  Constant6 : Constant  Priority=2
  Data Store Write1 : DataStoreWrite  Priority=4  DataStoreName=Tx_msg_count_CAN1
  Data Store Write2 : DataStoreWrite  Priority=4  DataStoreName=Tx_msg_count_CAN2
  wires:
  Constant6/1 -> Data Store Write1/1
  Constant1/1 -> Data Store Write2/1

== system HANcoder_E407_TTA_Controller_v3_2/HANcoder STM32 Target - E407-STM32 algorithm/TTA CAN System/TTA System/Matrix Cycle Manager/Controller Matrix Cycle/controller basic cycle 1/COMP Task - Rx_Sensor_Values_Check/Update Msg buffer ==
  note: If the msg received is coherent, we update the
      | stored copies of the set values. Otherwise, we
      | do not perform further calculations and raise an error.
  Enable : EnablePort
  Data Store Memory : DataStoreMemory  DataStoreName=mc_counter  ReadBeforeWriteMsg=warning  WriteAfterWriteMsg=warning  WriteAfterReadMsg=warning  InitialValue=1  ShowAdditionalParam=off
  Data Store Read2 : DataStoreRead  DataStoreName=mc_counter
  Data Store Read5 : DataStoreRead  DataStoreName=new_msg_Rx
  Data Store Read6 : DataStoreRead  DataStoreName=Msg_Rx
  NOT1 : Logic  Operator=NOT  IconShape=distinctive  AllPortsSameDT=off  OutDataTypeStr=boolean
  Sensor Values Rx Update : Subsystem  Priority=100  TreatAsAtomicUnit=on
  Sensor Values not Rx Update : Subsystem  Priority=110  TreatAsAtomicUnit=on
  Terminator : Terminator
  wires:
  Data Store Read5/1 -> Sensor Values Rx Update/Enable, NOT1/1  "new_sensor_rx_s"
  Data Store Read6/1 -> Sensor Values Rx Update/1(msg_rx)
  NOT1/1 -> Sensor Values not Rx Update/Enable
  Data Store Read2/1 -> Terminator/1  "mc_counter_s"

== system HANcoder_E407_TTA_Controller_v3_2/HANcoder STM32 Target - E407-STM32 algorithm/TTA CAN System/TTA System/Matrix Cycle Manager/Controller Matrix Cycle/controller basic cycle 1/COMP Task - Rx_Set_Values_Check/Process_Messages ==
  note: Logic Analyzer - DEBUG
  note: Logic Analyzer - DEBUG
      | Sync_Check COMP task
      | activation
  new_CAN1_msg : Inport
  new_CAN2_msg : Inport  Port=2
  Rx_msg_CAN1 : Inport  Port=3  OutDataTypeStr=Bus: msg_buffer_type
  Rx_Msg_CAN2 : Inport  Port=4  OutDataTypeStr=Bus: msg_buffer_type
  expected_board_id : Inport  Port=5
  Enable : EnablePort
  Bus Selector : BusSelector  OutputSignals=signal1,Buffer_2,Buffer_3,Buffer_4,Buffer_5,Buffer_6,Buffer_7,Buffer_8
  Constant2 : Constant  Priority=28  OutDataTypeStr=boolean
  Data Store Write : DataStoreWrite  Priority=4  DataStoreName=Msg_Rx  DataStoreElements=Msg_Rx.Buffer_1#Msg_Rx.Buffer_2#Msg_Rx.Buffer_3#Msg_Rx.Buffer_4#Msg_Rx.Buffer_5#Msg_Rx.Buffer_6#Msg_Rx.Buffer_7#Msg_Rx.Buffer_8
  Data Store Write1 : DataStoreWrite  DataStoreName=new_msg_Rx
  Data Store Write3 : DataStoreWrite  Priority=29  DataStoreName=Toggle_Pin_A0
  Demux message CAN1 and check coherence : Subsystem  Priority=1
  Demux message CAN1 and check coherence1 : Subsystem  Priority=2
  OR : Logic  Operator=OR  IconShape=distinctive  AllPortsSameDT=off  OutDataTypeStr=boolean
  Switch : Switch  Priority=3  Criteria=u2 > Threshold
  Terminator : Terminator
  Terminator1 : Terminator
  wires:
  Bus Selector/2 -> Data Store Write/2  "<Buffer_2>"
  Bus Selector/6 -> Data Store Write/6  "<Buffer_6>"
  Switch/1 -> Bus Selector/1
  Bus Selector/8 -> Data Store Write/8  "<Buffer_8>"
  Bus Selector/1 -> Data Store Write/1  "<signal1>"
  Bus Selector/7 -> Data Store Write/7  "<Buffer_7>"
  Bus Selector/4 -> Data Store Write/4  "<Buffer_4>"
  Bus Selector/3 -> Data Store Write/3  "<Buffer_3>"
  Bus Selector/5 -> Data Store Write/5  "<Buffer_5>"
  Demux message CAN1 and check coherence1/2(Msg_Count_CAN2) -> Terminator/1
  Demux message CAN1 and check coherence/2(Msg_Count_CAN1) -> Terminator1/1
  expected_board_id/1 -> Demux message CAN1 and check coherence1/2(expected_board_id), Demux message CAN1 and check coherence/2(expected_board_id)
  Constant2/1 -> Data Store Write3/1
  OR/1 -> Data Store Write1/1
  Demux message CAN1 and check coherence1/3(CAN2_msg) -> Switch/3
  Demux message CAN1 and check coherence1/1(CAN2_msg_coherent) -> OR/2
  Demux message CAN1 and check coherence/1(CAN1_msg) -> Switch/1
  Demux message CAN1 and check coherence/3(CAN1_msg_coherent) -> OR/1, Switch/2
  Rx_Msg_CAN2/1 -> Demux message CAN1 and check coherence1/1(CAN2_Rx_msg)
  Rx_msg_CAN1/1 -> Demux message CAN1 and check coherence/1(CAN1_Rx_msg)
  new_CAN2_msg/1 -> Demux message CAN1 and check coherence1/Enable
  new_CAN1_msg/1 -> Demux message CAN1 and check coherence/Enable

== system HANcoder_E407_TTA_Controller_v3_2/HANcoder STM32 Target - E407-STM32 algorithm/TTA CAN System/TTA System/Matrix Cycle Manager/Controller Matrix Cycle/controller basic cycle 1/COMP Task - Rx_Set_Values_Check/Reset Tx msg counter ==
  Enable : EnablePort
  Constant1 : Constant  Priority=2
  Constant6 : Constant  Priority=2
  Data Store Write1 : DataStoreWrite  Priority=4  DataStoreName=Tx_msg_count_CAN1
  Data Store Write2 : DataStoreWrite  Priority=4  DataStoreName=Tx_msg_count_CAN2
  wires:
  Constant1/1 -> Data Store Write2/1
  Constant6/1 -> Data Store Write1/1

== system HANcoder_E407_TTA_Controller_v3_2/HANcoder STM32 Target - E407-STM32 algorithm/TTA CAN System/TTA System/Matrix Cycle Manager/Controller Matrix Cycle/controller basic cycle 1/COMP Task - Rx_Set_Values_Check/Update Msg buffer ==
  note: If the msg received is coherent, we update the
      | stored copies of the set values. Otherwise, we
      | do not perform any more calculations and raise an error.
  Enable : EnablePort
  Data Store Read5 : DataStoreRead  DataStoreName=new_msg_Rx
  Data Store Read6 : DataStoreRead  DataStoreName=Msg_Rx
  NOT1 : Logic  Operator=NOT  IconShape=distinctive  AllPortsSameDT=off  OutDataTypeStr=boolean
  Set Values Update : Subsystem  Priority=100  TreatAsAtomicUnit=on
  Set Values not Rx : Subsystem  Priority=100  TreatAsAtomicUnit=on
  wires:
  NOT1/1 -> Set Values not Rx/Enable
  Data Store Read5/1 -> NOT1/1, Set Values Update/Enable  "new_set_rx_s"
  Data Store Read6/1 -> Set Values Update/1(msg_rx)

== system HANcoder_E407_TTA_Controller_v3_2/HANcoder STM32 Target - E407-STM32 algorithm/TTA CAN System/TTA System/Matrix Cycle Manager/Controller Matrix Cycle/controller basic cycle 1/COMP Task - Sync bc1 check/Process_Messages ==
  note: Logic Analyzer - DEBUG
      | Sync_Check COMP task
      | activation
  note: Logic Analyzer - DEBUG
  new_CAN1_msg : Inport
  new_CAN2_msg : Inport  Port=2
  Rx_msg_CAN1 : Inport  Port=3  OutDataTypeStr=Bus: msg_buffer_type
  Rx_Msg_CAN2 : Inport  Port=4  OutDataTypeStr=Bus: msg_buffer_type
  expected_basic_cycle : Inport  Port=5
  TM_COMM : Inport  Port=6
  expected_board_id : Inport  Port=7
  Enable : EnablePort
  Bus Selector : BusSelector  OutputSignals=signal1,Buffer_2,Buffer_3,Buffer_4,Buffer_5,Buffer_6,Buffer_7,Buffer_8
  Constant2 : Constant  Priority=28  OutDataTypeStr=boolean
  Data Store Write : DataStoreWrite  Priority=4  DataStoreName=Msg_Rx  DataStoreElements=Msg_Rx.Buffer_1#Msg_Rx.Buffer_2#Msg_Rx.Buffer_3#Msg_Rx.Buffer_4#Msg_Rx.Buffer_5#Msg_Rx.Buffer_6#Msg_Rx.Buffer_7#Msg_Rx.Buffer_8
  Data Store Write2 : DataStoreWrite  DataStoreName=new_msg_Rx
  Data Store Write3 : DataStoreWrite  Priority=29  DataStoreName=Toggle_Pin_A0
  Demux message CAN1 and check coherence : Subsystem  Priority=1
  Demux message CAN1 and check coherence1 : Subsystem  Priority=2
  Desync calculation : Subsystem  Priority=10
  OR : Logic  Operator=OR  IconShape=distinctive  AllPortsSameDT=off  OutDataTypeStr=boolean
  Switch : Switch  Priority=3  Criteria=u2 > Threshold
  wires:
  new_CAN1_msg/1 -> Demux message CAN1 and check coherence/Enable
  new_CAN2_msg/1 -> Demux message CAN1 and check coherence1/Enable
  Rx_msg_CAN1/1 -> Demux message CAN1 and check coherence/1(CAN1_Rx_msg)
  Rx_Msg_CAN2/1 -> Demux message CAN1 and check coherence1/1(CAN2_Rx_msg)
  Demux message CAN1 and check coherence/1(CAN1_msg) -> Switch/1
  Demux message CAN1 and check coherence1/1(CAN2_msg_coherent) -> OR/2
  Demux message CAN1 and check coherence1/3(CAN2_msg) -> Switch/3
  expected_basic_cycle/1 -> Demux message CAN1 and check coherence1/2(expected_basic_cycle), Demux message CAN1 and check coherence/2(expected_basic_cycle)
  Constant2/1 -> Data Store Write3/1
  expected_board_id/1 -> Demux message CAN1 and check coherence1/3(expected_board_id), Demux message CAN1 and check coherence/3(expected_board_id)
  Demux message CAN1 and check coherence/2(Msg_Count_CAN1) -> [msg_count_CAN1]
  Demux message CAN1 and check coherence1/2(Msg_Count_CAN2) -> [msg_count_CAN2]
  Switch/1 -> Bus Selector/1
  Bus Selector/1 -> Data Store Write/1  "<signal1>"
  Bus Selector/2 -> Data Store Write/2  "<Buffer_2>"
  Bus Selector/3 -> Data Store Write/3  "<Buffer_3>"
  Bus Selector/4 -> Data Store Write/4  "<Buffer_4>"
  Bus Selector/5 -> Data Store Write/5  "<Buffer_5>"
  Bus Selector/6 -> Data Store Write/6  "<Buffer_6>"
  Bus Selector/7 -> Data Store Write/7  "<Buffer_7>"
  Bus Selector/8 -> Data Store Write/8  "<Buffer_8>"
  [CAN1_msg_coherent_TAG] -> Desync calculation/2(New_msg_CAN1)
  Demux message CAN1 and check coherence/3(CAN1_msg_coherent) -> [CAN1_msg_coherent_TAG], Switch/2, OR/1
  [new_msg_Rx_TAG] -> Desync calculation/Enable
  OR/1 -> [new_msg_Rx_TAG], Data Store Write2/1
  TM_COMM/1 -> Desync calculation/1(TM_COMM)
  [msg_count_CAN1] -> Desync calculation/3(msg_count_CAN1)
  [msg_count_CAN2] -> Desync calculation/4(msg_count_CAN2)

== system HANcoder_E407_TTA_Controller_v3_2/HANcoder STM32 Target - E407-STM32 algorithm/TTA CAN System/TTA System/Matrix Cycle Manager/Controller Matrix Cycle/controller basic cycle 1/COMP Task - Sync bc1 check/Reset Tx msg counter ==
  Enable : EnablePort
  Constant1 : Constant  Priority=2
  Constant6 : Constant  Priority=2
  Data Store Write1 : DataStoreWrite  Priority=4  DataStoreName=Tx_msg_count_CAN1
  Data Store Write2 : DataStoreWrite  Priority=4  DataStoreName=Tx_msg_count_CAN2
  wires:
  Constant6/1 -> Data Store Write1/1
  Constant1/1 -> Data Store Write2/1
